simulink model "Radar"  (R2022b)
settings: Solver=FixedStepAuto  StartTime=0.0  StopTime=25  FixedStep=0.001  RelTol=1e-3
PreLoadFcn:
  | coder.extrinsic('plotPoints')
  | coder.extrinsic('MATLAB Function1')
libraries: fl_lib x11, simulink_extras x10, spsEdgeDetectorLib x8, nesl_utility x4, ee_lib x2, mcbresolverdecoderlib x1, simulink x1
settings Model: Creator=fercl  LastModifiedBy=fercl
settings DebuggingCC: UnderSpecifiedDimensionMsg=warning
settings ModelReferenceCC: EnableRefExpFcnMdlSchedulingChecks=on

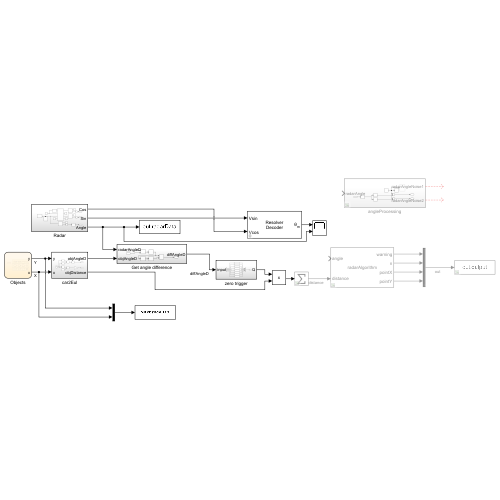
[thumbnail: Simulink's stored preview of the top-level diagram]
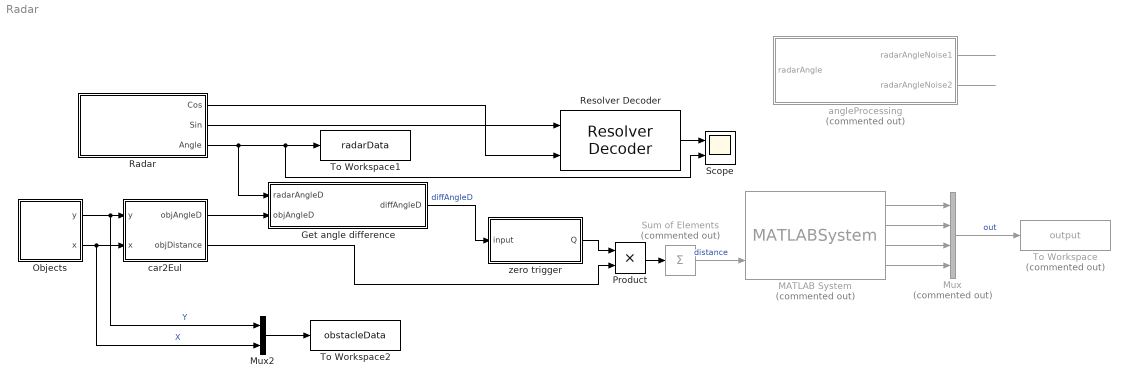
== system Radar ==
  Get angle difference : Subsystem
  MATLAB System : MATLABSystem  Commented=on  System=radarAlgorithm  radius=simParam.radius  distanceThreshold=simParam.threshold  SimulateUsing=Code generation
      mask Type: radarAlgorithm
      mask Display:
      | disp('radarAlgorithm');
      | port_label('input',1,'angle');
      | port_label('input',2,'distance');
      | port_label('output',1,'warning');
      | port_label('output',2,'n');
      | port_label('output',3,'pointX');
      | port_label('output',4,'pointY');
  Mux : Mux  Commented=on
  Mux2 : Mux  Inputs=2
  Objects : Stateflow chart  TreatAsAtomicUnit=on
  Product : Product
  Radar : Subsystem
  Resolver Decoder : mcbresolverdecoderlib/Resolver Decoder  MechPos=on  TrigElecPos=off  Speed=off  Pr=1  ExcitationMethod=Sinusoidal Excitation  Normilization=off  PhaseDelay=0.1746  SampleLength=16  Pm=3  RoundingMethod=Zero  BlockSampleTime=50e-6  PositionUnit=Degrees  SpeedUnit=Degrees/Sec  BaseSpeed=2000  DataTypeParameter=double  Offset=0
      settings: LibrarySourceBlock=mcblib/Sensor Decoders/Resolver Decoder
  Scope : Scope  NumInputPorts=2
  Sum of Elements : Sum  Commented=on  Inputs=+
  To Workspace : ToWorkspace  Commented=on  VariableName=output  SaveFormat=Timeseries  SampleTime=-1
  To Workspace1 : ToWorkspace  VariableName=radarData  SaveFormat=Timeseries  SampleTime=-1
  To Workspace2 : ToWorkspace  VariableName=obstacleData  SaveFormat=Timeseries  SampleTime=-1
  angleProcessing : Subsystem  Commented=on
  car2Eul : Subsystem
  zero trigger : Subsystem
  wires:
  Get angle difference/1(diffAngleD) -> zero trigger/1(input)  "diffAngleD"
  car2Eul/1(objAngleD) -> Get angle difference/2(objAngleD)
  zero trigger/1(Q) -> Product/1
  Sum of Elements/1 -> MATLAB System/2  "distance"
  car2Eul/2(objDistance) -> Product/2
  MATLAB System/1 -> Mux/1
  MATLAB System/2 -> Mux/2
  MATLAB System/3 -> Mux/3
  MATLAB System/4 -> Mux/4
  Mux/1 -> To Workspace/1  "out"
  Mux2/1 -> To Workspace2/1
  Objects/1(y) -> Mux2/1, car2Eul/1(y)  "Y"
  Objects/2(x) -> Mux2/2, car2Eul/2(x)  "X"
  Product/1 -> Sum of Elements/1
  angleProcessing/2(radarAngleNoise2) -> ?
  angleProcessing/1(radarAngleNoise1) -> ?
  Radar/3(Angle) -> Get angle difference/1(radarAngleD), Scope/2, To Workspace1/1
  Radar/2(Sin) -> Resolver Decoder/1
  Radar/1(Cos) -> Resolver Decoder/2
  Resolver Decoder/1 -> Scope/1

== system Radar/Get angle difference ==
  radarAngleD : Inport
  objAngleD : Inport  Port=2
  Abs : Abs  SaturateOnIntegerOverflow=off
  Abs1 : Abs  SaturateOnIntegerOverflow=off
  Add Constant : Bias  Bias=-360  SaturateOnIntegerOverflow=off
  Min1 : MinMax  Inputs=2
  Subtract : Sum  Inputs=+-
  diffAngleD : Outport
  wires:
  radarAngleD/1 -> Subtract/1
  Abs1/1 -> Min1/2
  objAngleD/1 -> Subtract/2
  Add Constant/1 -> Abs1/1
  Abs/1 -> Min1/1, Add Constant/1
  Subtract/1 -> Abs/1
  Min1/1 -> diffAngleD/1

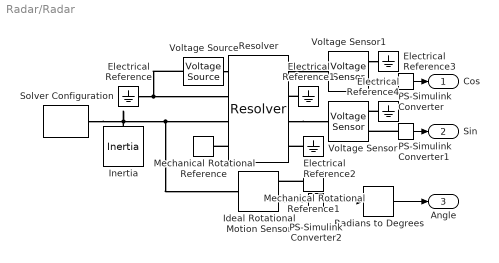
== system Radar/Radar ==
  Electrical Reference{,1..4} (5 alike) : fl_lib/Electrical/Electrical Elements/Electrical Reference
  Ideal Rotational Motion Sensor : fl_lib/Mechanical/Mechanical Sensors/Ideal Rotational Motion Sensor  reference=foundation.enum.MeasurementReference.difference  acceleration_port=false  velocity_port=false  position_port=true  wrap_angle=true  offset=0 rad
      settings: InternalSimscapePortConfiguration="{\"Bottom\":[],\"Left\":[{\"id\":\"R\",\"label\":\"R\",\"type\":\"foundation.mechanical.rotational.rotational\"}],\"Right\":[{\"id\":\"C\",\"label\":\"C\",\"type\":\"foundation.mechanical.rotational.rotational\"},{\"id\":\"A\",\"label\":\"A\",\"type\":\"output\"}],\"Top\":[]}"
  Inertia : fl_lib/Mechanical/Rotational Elements/Inertia  inertia=0.01 kg*m^2  num_ports=foundation.enum.numPorts2.one  w_specify=on  w_priority=High  w=60 rpm  w_nominal_specify=off  w_nominal_unit=rad/s  w_nominal_value=1  t_specify=off  t_priority=None  t=0 N*m  t_nominal_specify=off  t_nominal_unit=N*m  t_nominal_value=1
  Mechanical Rotational Reference : fl_lib/Mechanical/Rotational Elements/Mechanical Rotational Reference
  Mechanical Rotational Reference1 : fl_lib/Mechanical/Rotational Elements/Mechanical Rotational Reference
  PS-Simulink Converter : nesl_utility/PS-Simulink Converter  PhysicalDomain=network_engine_domain  SubClassName=ps_output  LeftPortType=input  RightPortType=output  PseudoPeriodic=off  Frequencies=[]  VectorFormat=inherit  Unit=inherit  AffineConversion=off
  PS-Simulink Converter1 : nesl_utility/PS-Simulink Converter  PhysicalDomain=network_engine_domain  SubClassName=ps_output  LeftPortType=input  RightPortType=output  PseudoPeriodic=off  Frequencies=[]  VectorFormat=inherit  Unit=inherit  AffineConversion=off
  PS-Simulink Converter2 : nesl_utility/PS-Simulink Converter  PhysicalDomain=network_engine_domain  SubClassName=ps_output  LeftPortType=input  RightPortType=output  PseudoPeriodic=off  Frequencies=[]  VectorFormat=inherit  Unit=inherit  AffineConversion=off
  Radians to Degrees : simulink_extras/Transformations/Radians to Degrees
  Resolver : ee_lib/Sensors & Transducers/Resolver  parameterization=1  ratio=0.5  Rr=70 Ohm  Rs=180 Ohm  Xr=100 Ohm  Xs=300 Ohm  omega=10 kHz  Lr=0.0016 H  Ls=0.0048 H  k=0.35  N=1  theta_specify=off  theta_priority=High  theta=0 deg  theta_nominal_specify=off  theta_nominal_unit=deg  theta_nominal_value=1
      settings: InternalSimscapePortConfiguration="{\"Bottom\":[],\"Left\":[{\"id\":\"p1\",\"label\":\"p1\",\"type\":\"foundation.electrical.electrical\"},{\"id\":\"p2\",\"label\":\"p2\",\"type\":\"foundation.electrical.electrical\"},{\"id\":\"R\",\"label\":\"R\",\"type\":\"foundation.mechanical.rotational.rotational\"},{\"id\":\"C\",\"label\":\"C\",\"type\":\"foundation.mechanical.rotational.rotational\"}],\"Right\":[{\"id\":\"x1\",\"label\":\"x1\",\"type\":\"foundation.electrical.electrical\"},{\"id\":\"x2\",\"label\":\"x2\",\"type\":\"foundation.electrical.electrical\"},{\"id\":\"y1\",\"label\":\"y1\",\"type\":\"foundation.electrical.electrical\"},{\"id\":\"y2\",\"label\":\"y2\",\"type\":\"foundation.electrical.electrical\"}],\"Top\":[]}"
  Solver Configuration : nesl_utility/Solver Configuration  PhysicalDomain=network_engine_domain  SubClassName=solver  LeftPortType=input  RightPortType=generic  Tones=[]  Harmonics=[]  SimulateNoise=off  Profile=off  UseLocalSampling=off  EnableSwitchedLinearOptims=on  FrequencyDomain=off  UseCCode=off  RelTol=0.001  AbsTol=0.001  MinStep=1e-09  ToWorkspace=off  RevertToSquareIcSolve=off  NumHomotopyIterations=100  PhasorMode=off  PhasorModeNumHarmonics=1  ConsistencySolver=NEWTON_XTOL_AFTER_FTOL  IndexReductionMethod=DerivativeReplacement  DoDC=off  ResidualTolerance=1e-09  ConsistencyTolSource=GLOBAL  ConsistencyAbsTol=0.001  ConsistencyRelTol=0.001  ConsistencyTolFactor=0.001  UseLocalSolver=off  LocalSolverChoice=NE_BACKWARD_EULER_ADVANCER  ResolveIndetEquations=on  FunctionEvalNumThread=1  LocalSolverSampleTime=0.001  DoFixedCost=off  MaxNonlinIter=3  MaxModeIter=2  ComputeImpulses=off  ImpulseIterations=2  LinearAlgebra=auto  LinearAlgebraNumThread=0  EquationFormulation=NE_TIME_EF  DelaysMemoryBudget=1024  AutomaticFiltering=on  FilteringTimeConstant=0.001  PartitionStorageMethod=AS_NEEDED  PartitionMemoryBudget=1024  PartitionMethod=ROBUST
  Voltage Sensor : fl_lib/Electrical/Electrical Sensors/Voltage Sensor
  Voltage Sensor1 : fl_lib/Electrical/Electrical Sensors/Voltage Sensor
  Voltage Source : ee_lib/Sources/Voltage Source  dc_voltage=0 V  ac_voltage=1 V  ac_shift=0 rad  ac_frequency=400 Hz  noise_mode=ee.enum.sources.noise.Disabled  PSD=0 V^2/Hz  sample_time=1e-3 s  repeatability=ee.enum.sources.repeatability.NotRepeatable  user_seed=0  auto_seed=545404223  i_specify=off  i_priority=None  i=0 A  i_nominal_specify=off  i_nominal_unit=A  i_nominal_value=1  v_specify=off  v_priority=None  v=0 V  v_nominal_specify=off  v_nominal_unit=V  v_nominal_value=1
  Cos : Outport
  Sin : Outport  Port=2
  Angle : Outport  Port=3
  wires:
  PS-Simulink Converter/1 -> Cos/1
  PS-Simulink Converter1/1 -> Sin/1
  PS-Simulink Converter2/1 -> Radians to Degrees/1
  Radians to Degrees/1 -> Angle/1
  connections:
  Inertia/LConn1 -- Solver Configuration/RConn1 -- Ideal Rotational Motion Sensor/LConn1 -- Resolver/LConn3
  Resolver/LConn4 -- Mechanical Rotational Reference/LConn1
  Voltage Source/LConn1 -- Resolver/LConn1
  Voltage Source/RConn1 -- Electrical Reference/LConn1 -- Resolver/LConn2
  Resolver/RConn3 -- Voltage Sensor/LConn1
  Resolver/RConn1 -- Voltage Sensor1/LConn1
  PS-Simulink Converter/LConn1 -- Voltage Sensor1/RConn1
  Electrical Reference1/LConn1 -- Resolver/RConn2
  Electrical Reference2/LConn1 -- Resolver/RConn4
  Voltage Sensor1/RConn2 -- Electrical Reference3/LConn1
  Electrical Reference4/LConn1 -- Voltage Sensor/RConn2
  PS-Simulink Converter1/LConn1 -- Voltage Sensor/RConn1
  Mechanical Rotational Reference1/LConn1 -- Ideal Rotational Motion Sensor/RConn1
  Ideal Rotational Motion Sensor/RConn2 -- PS-Simulink Converter2/LConn1

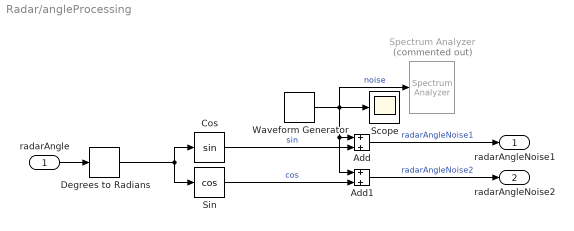
== system Radar/angleProcessing ==
  radarAngle : Inport
  Add : Sum
  Add1 : Sum
  Cos : Trigonometry
  Degrees to Radians : simulink_extras/Transformations/Degrees to Radians
  Scope : Scope
  Sin : Trigonometry  Operator=cos
  Spectrum Analyzer : SpectrumAnalyzer  Commented=on
  Waveform Generator : simulink/Sources/Waveform Generator  OutMin=[]  OutMax=[]  OutDataTypeStr=double  SelectedSignal=1  Signals=sin(0.1, 50*2*pi, 0)+sin(0.1, 75*2*pi, 0)+sin(0.1, 100*2*pi, 0)  BlockNames=MultiportSwitch_22b4aa63d103428  SampleTime=0.001
  radarAngleNoise1 : Outport
  radarAngleNoise2 : Outport  Port=2
  wires:
  radarAngle/1 -> Degrees to Radians/1
  Cos/1 -> Add/2  "sin"
  Waveform Generator/1 -> Spectrum Analyzer/1, Scope/1, Add1/1, Add/1  "noise"
  Sin/1 -> Add1/2  "cos"
  Add1/1 -> radarAngleNoise2/1  "radarAngleNoise2"
  Add/1 -> radarAngleNoise1/1  "radarAngleNoise1"
  Degrees to Radians/1 -> Sin/1, Cos/1

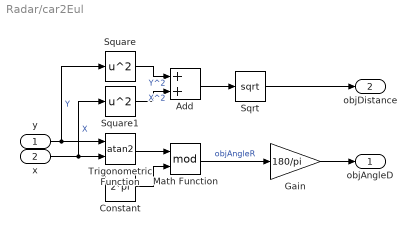
== system Radar/car2Eul ==
  y : Inport
  x : Inport  Port=2
  Add : Sum
  Constant : Constant  Value=2*pi
  Gain : Gain  Gain=180/pi
  Math Function : Math  Operator=mod
  Sqrt : Sqrt
  Square : Math  Operator=square
  Square1 : Math  Operator=square
  Trigonometric Function : Trigonometry  Operator=atan2
  objAngleD : Outport
  objDistance : Outport  Port=2
  wires:
  Constant/1 -> Math Function/2
  x/1 -> Square1/1, Trigonometric Function/2  "X"
  Trigonometric Function/1 -> Math Function/1
  Math Function/1 -> Gain/1  "objAngleR"
  y/1 -> Square/1, Trigonometric Function/1  "Y"
  Gain/1 -> objAngleD/1
  Square/1 -> Add/1  "Y^2"
  Square1/1 -> Add/2  "X^2"
  Add/1 -> Sqrt/1
  Sqrt/1 -> objDistance/1

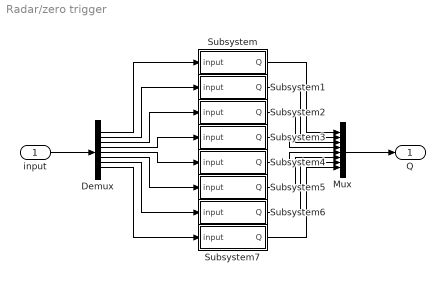
== system Radar/zero trigger ==
  input : Inport
  Demux : Demux  Outputs=8
  Mux : Mux  Inputs=8
  Subsystem : Subsystem
  Subsystem1 : Subsystem
  Subsystem2 : Subsystem
  Subsystem3 : Subsystem
  Subsystem4 : Subsystem
  Subsystem5 : Subsystem
  Subsystem6 : Subsystem
  Subsystem7 : Subsystem
  Q : Outport
  wires:
  input/1 -> Demux/1
  Demux/1 -> Subsystem/1(input)
  Demux/2 -> Subsystem1/1(input)
  Demux/3 -> Subsystem2/1(input)
  Demux/4 -> Subsystem3/1(input)
  Demux/5 -> Subsystem4/1(input)
  Demux/6 -> Subsystem5/1(input)
  Demux/7 -> Subsystem6/1(input)
  Demux/8 -> Subsystem7/1(input)
  Subsystem/1(Q) -> Mux/1
  Subsystem1/1(Q) -> Mux/2
  Subsystem2/1(Q) -> Mux/3
  Subsystem3/1(Q) -> Mux/4
  Subsystem4/1(Q) -> Mux/5
  Subsystem5/1(Q) -> Mux/6
  Subsystem6/1(Q) -> Mux/7
  Subsystem7/1(Q) -> Mux/8
  Mux/1 -> Q/1

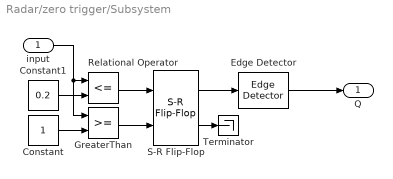
== system Radar/zero trigger/Subsystem ==
  input : Inport
  Constant : Constant
  Constant1 : Constant  Value=0.2
  Edge Detector : spsEdgeDetectorLib/Edge Detector  model=Rising  ic=0  Ts=0
      settings: LibrarySourceBlock=sps_lib/Control/Edge Detector
  GreaterThan : RelationalOperator  OutDataTypeStr=boolean  RndMeth=Simplest  InputSameDT=off
  Relational Operator : RelationalOperator  Operator=<=  OutDataTypeStr=boolean  RndMeth=Simplest  InputSameDT=off
  S-R Flip-Flop : simulink_extras/Flip Flops/S-R Flip-Flop  initial_condition=0
  Terminator : Terminator
  Q : Outport
  wires:
  S-R Flip-Flop/1 -> Edge Detector/1
  input/1 -> GreaterThan/1, Relational Operator/1
  S-R Flip-Flop/2 -> Terminator/1
  Edge Detector/1 -> Q/1
  Relational Operator/1 -> S-R Flip-Flop/1
  Constant/1 -> GreaterThan/2
  Constant1/1 -> Relational Operator/2
  GreaterThan/1 -> S-R Flip-Flop/2

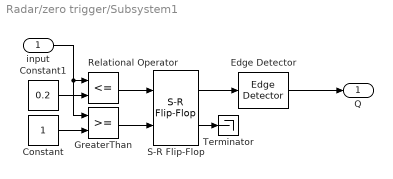
== system Radar/zero trigger/Subsystem1 ==
  input : Inport
  Constant : Constant
  Constant1 : Constant  Value=0.2
  Edge Detector : spsEdgeDetectorLib/Edge Detector  model=Rising  ic=0  Ts=0
      settings: LibrarySourceBlock=sps_lib/Control/Edge Detector
  GreaterThan : RelationalOperator  OutDataTypeStr=boolean  RndMeth=Simplest  InputSameDT=off
  Relational Operator : RelationalOperator  Operator=<=  OutDataTypeStr=boolean  RndMeth=Simplest  InputSameDT=off
  S-R Flip-Flop : simulink_extras/Flip Flops/S-R Flip-Flop  initial_condition=0
  Terminator : Terminator
  Q : Outport
  wires:
  S-R Flip-Flop/1 -> Edge Detector/1
  input/1 -> GreaterThan/1, Relational Operator/1
  S-R Flip-Flop/2 -> Terminator/1
  Edge Detector/1 -> Q/1
  Relational Operator/1 -> S-R Flip-Flop/1
  Constant/1 -> GreaterThan/2
  Constant1/1 -> Relational Operator/2
  GreaterThan/1 -> S-R Flip-Flop/2

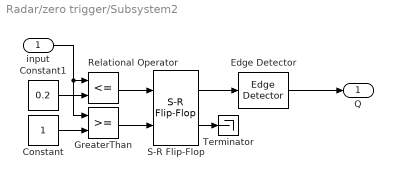
== system Radar/zero trigger/Subsystem2 ==
  input : Inport
  Constant : Constant
  Constant1 : Constant  Value=0.2
  Edge Detector : spsEdgeDetectorLib/Edge Detector  model=Rising  ic=0  Ts=0
      settings: LibrarySourceBlock=sps_lib/Control/Edge Detector
  GreaterThan : RelationalOperator  OutDataTypeStr=boolean  RndMeth=Simplest  InputSameDT=off
  Relational Operator : RelationalOperator  Operator=<=  OutDataTypeStr=boolean  RndMeth=Simplest  InputSameDT=off
  S-R Flip-Flop : simulink_extras/Flip Flops/S-R Flip-Flop  initial_condition=0
  Terminator : Terminator
  Q : Outport
  wires:
  S-R Flip-Flop/1 -> Edge Detector/1
  input/1 -> GreaterThan/1, Relational Operator/1
  S-R Flip-Flop/2 -> Terminator/1
  Edge Detector/1 -> Q/1
  Relational Operator/1 -> S-R Flip-Flop/1
  Constant/1 -> GreaterThan/2
  Constant1/1 -> Relational Operator/2
  GreaterThan/1 -> S-R Flip-Flop/2

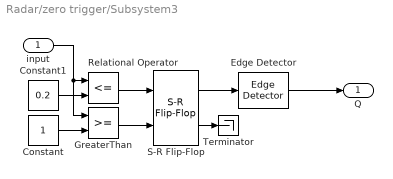
== system Radar/zero trigger/Subsystem3 ==
  input : Inport
  Constant : Constant
  Constant1 : Constant  Value=0.2
  Edge Detector : spsEdgeDetectorLib/Edge Detector  model=Rising  ic=0  Ts=0
      settings: LibrarySourceBlock=sps_lib/Control/Edge Detector
  GreaterThan : RelationalOperator  OutDataTypeStr=boolean  RndMeth=Simplest  InputSameDT=off
  Relational Operator : RelationalOperator  Operator=<=  OutDataTypeStr=boolean  RndMeth=Simplest  InputSameDT=off
  S-R Flip-Flop : simulink_extras/Flip Flops/S-R Flip-Flop  initial_condition=0
  Terminator : Terminator
  Q : Outport
  wires:
  S-R Flip-Flop/1 -> Edge Detector/1
  input/1 -> GreaterThan/1, Relational Operator/1
  S-R Flip-Flop/2 -> Terminator/1
  Edge Detector/1 -> Q/1
  Relational Operator/1 -> S-R Flip-Flop/1
  Constant/1 -> GreaterThan/2
  Constant1/1 -> Relational Operator/2
  GreaterThan/1 -> S-R Flip-Flop/2

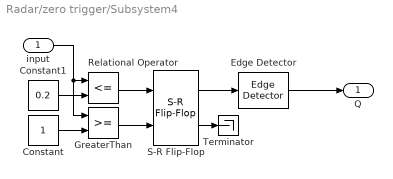
== system Radar/zero trigger/Subsystem4 ==
  input : Inport
  Constant : Constant
  Constant1 : Constant  Value=0.2
  Edge Detector : spsEdgeDetectorLib/Edge Detector  model=Rising  ic=0  Ts=0
      settings: LibrarySourceBlock=sps_lib/Control/Edge Detector
  GreaterThan : RelationalOperator  OutDataTypeStr=boolean  RndMeth=Simplest  InputSameDT=off
  Relational Operator : RelationalOperator  Operator=<=  OutDataTypeStr=boolean  RndMeth=Simplest  InputSameDT=off
  S-R Flip-Flop : simulink_extras/Flip Flops/S-R Flip-Flop  initial_condition=0
  Terminator : Terminator
  Q : Outport
  wires:
  S-R Flip-Flop/1 -> Edge Detector/1
  input/1 -> GreaterThan/1, Relational Operator/1
  S-R Flip-Flop/2 -> Terminator/1
  Edge Detector/1 -> Q/1
  Relational Operator/1 -> S-R Flip-Flop/1
  Constant/1 -> GreaterThan/2
  Constant1/1 -> Relational Operator/2
  GreaterThan/1 -> S-R Flip-Flop/2

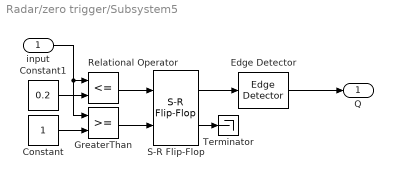
== system Radar/zero trigger/Subsystem5 ==
  input : Inport
  Constant : Constant
  Constant1 : Constant  Value=0.2
  Edge Detector : spsEdgeDetectorLib/Edge Detector  model=Rising  ic=0  Ts=0
      settings: LibrarySourceBlock=sps_lib/Control/Edge Detector
  GreaterThan : RelationalOperator  OutDataTypeStr=boolean  RndMeth=Simplest  InputSameDT=off
  Relational Operator : RelationalOperator  Operator=<=  OutDataTypeStr=boolean  RndMeth=Simplest  InputSameDT=off
  S-R Flip-Flop : simulink_extras/Flip Flops/S-R Flip-Flop  initial_condition=0
  Terminator : Terminator
  Q : Outport
  wires:
  S-R Flip-Flop/1 -> Edge Detector/1
  input/1 -> GreaterThan/1, Relational Operator/1
  S-R Flip-Flop/2 -> Terminator/1
  Edge Detector/1 -> Q/1
  Relational Operator/1 -> S-R Flip-Flop/1
  Constant/1 -> GreaterThan/2
  Constant1/1 -> Relational Operator/2
  GreaterThan/1 -> S-R Flip-Flop/2

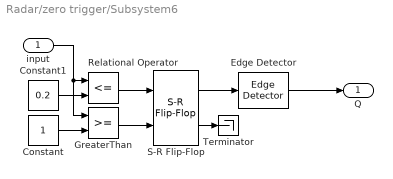
== system Radar/zero trigger/Subsystem6 ==
  input : Inport
  Constant : Constant
  Constant1 : Constant  Value=0.2
  Edge Detector : spsEdgeDetectorLib/Edge Detector  model=Rising  ic=0  Ts=0
      settings: LibrarySourceBlock=sps_lib/Control/Edge Detector
  GreaterThan : RelationalOperator  OutDataTypeStr=boolean  RndMeth=Simplest  InputSameDT=off
  Relational Operator : RelationalOperator  Operator=<=  OutDataTypeStr=boolean  RndMeth=Simplest  InputSameDT=off
  S-R Flip-Flop : simulink_extras/Flip Flops/S-R Flip-Flop  initial_condition=0
  Terminator : Terminator
  Q : Outport
  wires:
  S-R Flip-Flop/1 -> Edge Detector/1
  input/1 -> GreaterThan/1, Relational Operator/1
  S-R Flip-Flop/2 -> Terminator/1
  Edge Detector/1 -> Q/1
  Relational Operator/1 -> S-R Flip-Flop/1
  Constant/1 -> GreaterThan/2
  Constant1/1 -> Relational Operator/2
  GreaterThan/1 -> S-R Flip-Flop/2

== system Radar/zero trigger/Subsystem7 ==
  input : Inport
  Constant : Constant
  Constant1 : Constant  Value=0.2
  Edge Detector : spsEdgeDetectorLib/Edge Detector  model=Rising  ic=0  Ts=0
      settings: LibrarySourceBlock=sps_lib/Control/Edge Detector
  GreaterThan : RelationalOperator  OutDataTypeStr=boolean  RndMeth=Simplest  InputSameDT=off
  Relational Operator : RelationalOperator  Operator=<=  OutDataTypeStr=boolean  RndMeth=Simplest  InputSameDT=off
  S-R Flip-Flop : simulink_extras/Flip Flops/S-R Flip-Flop  initial_condition=0
  Terminator : Terminator
  Q : Outport
  wires:
  S-R Flip-Flop/1 -> Edge Detector/1
  input/1 -> GreaterThan/1, Relational Operator/1
  S-R Flip-Flop/2 -> Terminator/1
  Edge Detector/1 -> Q/1
  Relational Operator/1 -> S-R Flip-Flop/1
  Constant/1 -> GreaterThan/2
  Constant1/1 -> Relational Operator/2
  GreaterThan/1 -> S-R Flip-Flop/2

== stateflow chart Radar/Objects ==
  state Object1 [parallel]
    settings: executionOrder=2
    state O1MoveRight
      during:
      x(1) = x(1) + 0.001;
      exit:
      x(1) = x(1) + 0.001;
    state O1MoveDown
      during:
      y(1) = y(1) - 0.001;
      exit:
      y(1) = y(1) - 0.001;
    state O1MoveUpLeft
      during:
      y(1) = y(1) + 0.001;
      x(1) = x(1) - 0.001;
      exit:
      y(1) = y(1) + 0.001;
      x(1) = x(1) - 0.001;
    state O1Stop
    (default) -> O1MoveRight : {x(1) = 5; y(1) = 0;}
    O1MoveRight -> O1MoveDown : after(5,sec)
    O1MoveDown -> O1MoveUpLeft : after(5,sec)
    O1MoveUpLeft -> O1Stop : after(10,sec)
  state Reset [parallel]
    entry:
    x(1:8) = 0;
    y(1:8) = 0;
    settings: executionOrder=1
  state Object2 [parallel]
    settings: executionOrder=3
    state O2MoveLeft
      during:
      x(2) = x(2) - 0.001;
      exit:
      x(2) = x(2) - 0.001;
    state O2MoveUp
      during:
      y(2) = y(2) + 0.001;
      exit:
      y(2) = y(2) + 0.001;
    state O2MoveDownRight
      during:
      y(2) = y(2) - 0.001;
      x(2) = x(2) + 0.001;
      exit:
      y(2) = y(2) - 0.001;
      x(2) = x(2) + 0.001;
    state O2Stop
    (default) -> O2MoveLeft : {x(2) = -5; y(2) = 0;}
    O2MoveLeft -> O2MoveUp : after(5,sec)
    O2MoveUp -> O2MoveDownRight : after(5,sec)
    O2MoveDownRight -> O2Stop : after(10,sec)
  state Object3 [parallel]
    settings: executionOrder=4
    state O3MoveLeft
      during:
      x(3) = x(3) + 0.003;
      exit:
      x(3) = x(3) + 0.003;
    state O3MoveUp
      during:
      y(3) = y(3) - 0.003;
      exit:
      y(3) = y(3) - 0.003;
    state O3MoveDownRight
      during:
      x(3) = x(3) - 0.003;
      exit:
      x(3) = x(3) - 0.003;
    state O3Stop
    (default) -> O3MoveLeft : {x(3) = -15; y(3) = 15;}
    O3MoveLeft -> O3MoveUp : after(10,sec)
    O3MoveUp -> O3MoveDownRight : after(10,sec)
    O3MoveDownRight -> O3Stop : after(5,sec)
  data: y output size=[1 8] =0; x output size=[1 8] =0
